simulink model "P_Control"  (R2024b)
settings: Solver=VariableStepAuto  StartTime=0.0  StopTime=time  RelTol=1e-3
values from neighbouring files (symbols this model uses):
  As = 2.15    [Data.m]
  B = (y1-y4)/2    (= 0.75)    [Data.m]
  Cd = 0.28    [Data.m]
  clockwise = 1    [Data.m]
  dd = 2    [Data.m]
  delay_Pulse_time = 1.5    [Data.m]
  derta1 = 0.5    [Data.m]
  dk = 2    [Data.m]
  Fi = Ti/r    (= 156.25)    [Data.m]
  Fz = la/(la+lb)*m*g/2    (= 2450)    [Data.m]
  id = 0.01    [Data.m]
  ik = 1    [Data.m]
  Iw = 0.5    [Data.m]
  Iz = 1600    [Data.m]
  JL = 0.08    [Data.m]
  Jm = 6.96e-6    (= 6.96e-06)    [Data.m]
  Kb = 0.0525    [Data.m]
  Kf = 1.4e-3    (= 0.0014)    [Data.m]
  Km = 0.053    [Data.m]
  L = 6.2e-4    (= 0.00062)    [Data.m]    (also in submit.m = (1-nameda1)*(1-0.015*u1*sqrt((cx^2)*(nameda1^2)+(cy^2)*((tan)
  la = x1    (= 1.25)    [Data.m]
  lb = x1    (= 1.25)    [Data.m]
  m = 1000    [Data.m]
  modeli = 1    [Data.m]
  n = 1/200    (= 0.005)    [Data.m]
  pd = 100    [Data.m]
  pk = 300    [Data.m]
  Pulse = 180    [Data.m]
  R = 2.07    [Data.m]
  r = 0.32    [Data.m]
  s_ang3 = 0    [Data.m]
  x1 = 1.25    [Data.m]
  x1_fc = 0.01    [Data.m]
  x1_jz = 0    [Data.m]
  x2 = -1.25    [Data.m]
  x2_fc = 0.05    [Data.m]
  x2_jz = 0.01    [Data.m]
  x3 = -1.25    [Data.m]
  x3_fc = 0.1    [Data.m]
  x3_jz = 0.05    [Data.m]
  x4 = 1.25    [Data.m]
  x4_fc = 0.5    [Data.m]
  x4_jz = 0.08    [Data.m]
  Xicr = 0,Yicr=10    [Data.m]
  y1 = 0.75    [Data.m]
  y2 = 0.75    [Data.m]
  y3 = -0.75    [Data.m]
  y4 = -0.75    [Data.m]
undefined symbols (not defined in the file or in its folder): Yicr
libraries: slpidlib x12
(part 2 of 2)

== system P_Control/Subsystem1/电机模型5 ==
  电流1 : Inport
  干扰 : Inport  Port=2
  Add : Sum
  Add1 : Sum  Inputs=+-
  Add2 : Sum
  Constant : Constant  Value=s_ang3
  Constant1 : Constant  Value=(Jm+n^2*JL)
  Divide : Product  Inputs=*/
  Gain3 : Gain  Gain=n*Km
  Gain4 : Gain  Gain=Kf
  Gain5 : Gain  Gain=n^2
  Integrator : Integrator
  Integrator1 : Integrator  InitialCondition=0.01
  输出转角 : Outport
  wires:
  Add2/1 -> Divide/1
  Add1/1 -> Add2/2
  Gain5/1 -> Add2/1
  Gain4/1 -> Add1/2
  Gain3/1 -> Add1/1
  Constant1/1 -> Divide/2
  Divide/1 -> Integrator1/1
  Integrator1/1 -> Gain4/1, Integrator/1
  干扰/1 -> Gain5/1
  电流1/1 -> Gain3/1
  Add/1 -> 输出转角/1
  Integrator/1 -> Add/2
  Constant/1 -> Add/1

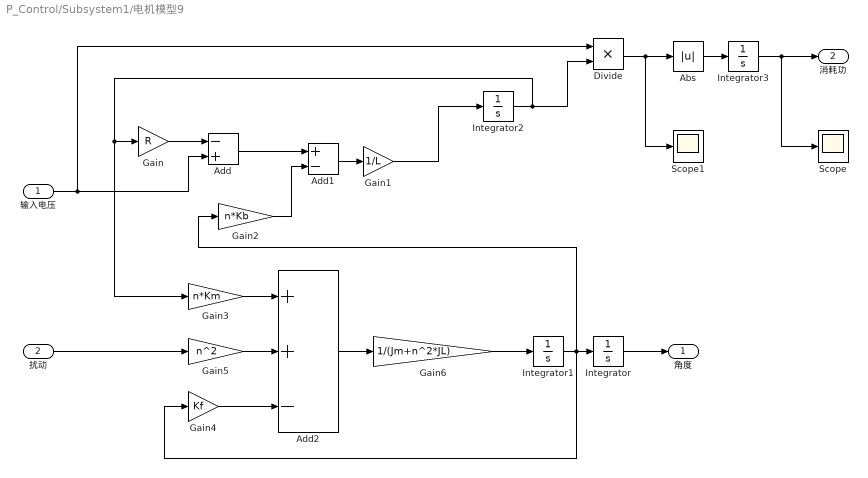
== system P_Control/Subsystem1/电机模型9 ==
  输入电压 : Inport
  扰动 : Inport  Port=2
  Abs : Abs  ZeroCross=off  SaturateOnIntegerOverflow=off
  Add : Sum  Inputs=-+
  Add1 : Sum  Inputs=+-
  Add2 : Sum  Inputs=++-
  Divide : Product  Inputs=**
  Gain : Gain  Gain=R
  Gain1 : Gain  Gain=1/L
  Gain2 : Gain  Gain=n*Kb
  Gain3 : Gain  Gain=n*Km
  Gain4 : Gain  Gain=Kf
  Gain5 : Gain  Gain=n^2
  Gain6 : Gain  Gain=1/(Jm+n^2*JL)
  Integrator{,1..3} (4 alike) : Integrator
  Scope : Scope
  Scope1 : Scope
  角度 : Outport
  消耗功 : Outport  Port=2
  wires:
  Divide/1 -> Scope1/1, Abs/1
  Gain6/1 -> Integrator1/1
  Add2/1 -> Gain6/1
  Gain4/1 -> Add2/3
  Gain5/1 -> Add2/2
  Gain3/1 -> Add2/1
  扰动/1 -> Gain5/1
  Gain1/1 -> Integrator2/1
  Add1/1 -> Gain1/1
  Gain2/1 -> Add1/2
  Add/1 -> Add1/1
  输入电压/1 -> Add/2, Divide/1
  Gain/1 -> Add/1
  Integrator2/1 -> Divide/2, Gain/1, Gain3/1
  Integrator1/1 -> Integrator/1, Gain4/1, Gain2/1
  Integrator/1 -> 角度/1
  Abs/1 -> Integrator3/1
  Integrator3/1 -> 消耗功/1, Scope/1

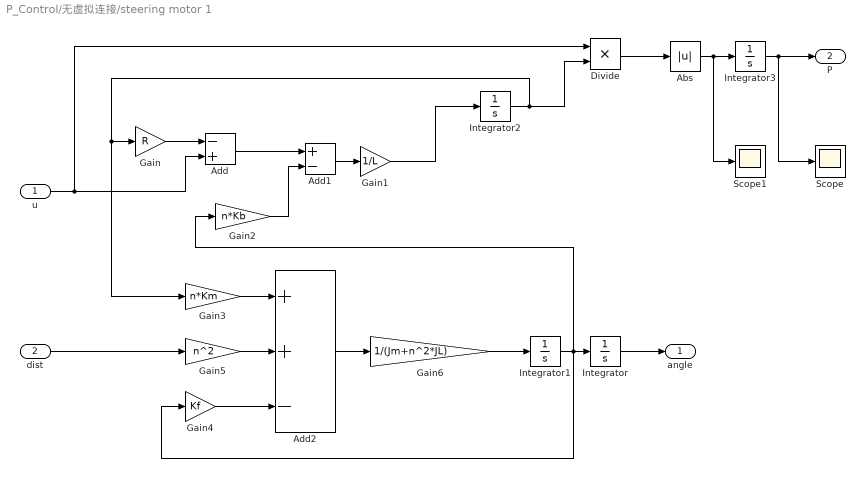
== system P_Control/无虚拟连接/steering motor 1 ==
  u : Inport
  dist : Inport  Port=2
  Abs : Abs  SaturateOnIntegerOverflow=off
  Add : Sum  Inputs=-+
  Add1 : Sum  Inputs=+-
  Add2 : Sum  Inputs=++-
  Divide : Product  Inputs=**
  Gain : Gain  Gain=R
  Gain1 : Gain  Gain=1/L
  Gain2 : Gain  Gain=n*Kb
  Gain3 : Gain  Gain=n*Km
  Gain4 : Gain  Gain=Kf
  Gain5 : Gain  Gain=n^2
  Gain6 : Gain  Gain=1/(Jm+n^2*JL)
  Integrator{,1..3} (4 alike) : Integrator
  Scope : Scope
  Scope1 : Scope
  angle : Outport
  P : Outport  Port=2
  wires:
  Integrator3/1 -> P/1, Scope/1
  Abs/1 -> Scope1/1, Integrator3/1
  Divide/1 -> Abs/1
  Gain6/1 -> Integrator1/1
  Add2/1 -> Gain6/1
  Gain4/1 -> Add2/3
  Gain5/1 -> Add2/2
  Gain3/1 -> Add2/1
  dist/1 -> Gain5/1
  Gain1/1 -> Integrator2/1
  Add1/1 -> Gain1/1
  Gain2/1 -> Add1/2
  Add/1 -> Add1/1
  u/1 -> Add/2, Divide/1
  Gain/1 -> Add/1
  Integrator2/1 -> Divide/2, Gain/1, Gain3/1
  Integrator1/1 -> Integrator/1, Gain4/1, Gain2/1
  Integrator/1 -> angle/1

== system P_Control/无虚拟连接/steering motor 2 ==
  u : Inport
  dist : Inport  Port=2
  Abs : Abs  SaturateOnIntegerOverflow=off
  Add : Sum  Inputs=-+
  Add1 : Sum  Inputs=+-
  Add2 : Sum  Inputs=++-
  Divide : Product  Inputs=**
  Gain : Gain  Gain=R
  Gain1 : Gain  Gain=1/L
  Gain2 : Gain  Gain=n*Kb
  Gain3 : Gain  Gain=n*Km
  Gain4 : Gain  Gain=Kf
  Gain5 : Gain  Gain=n^2
  Gain6 : Gain  Gain=1/(Jm+n^2*JL)
  Integrator{,1..3} (4 alike) : Integrator
  Scope : Scope
  angle : Outport
  P : Outport  Port=2
  wires:
  Integrator3/1 -> P/1, Scope/1
  Abs/1 -> Integrator3/1
  Divide/1 -> Abs/1
  Gain6/1 -> Integrator1/1
  Add2/1 -> Gain6/1
  Gain4/1 -> Add2/3
  Gain5/1 -> Add2/2
  Gain3/1 -> Add2/1
  dist/1 -> Gain5/1
  Gain1/1 -> Integrator2/1
  Add1/1 -> Gain1/1
  Gain2/1 -> Add1/2
  Add/1 -> Add1/1
  u/1 -> Add/2, Divide/1
  Gain/1 -> Add/1
  Integrator2/1 -> Divide/2, Gain/1, Gain3/1
  Integrator1/1 -> Integrator/1, Gain4/1, Gain2/1
  Integrator/1 -> angle/1

== system P_Control/无虚拟连接/steering motor 3 ==
  u : Inport
  dist : Inport  Port=2
  Abs : Abs  SaturateOnIntegerOverflow=off
  Add : Sum  Inputs=-+
  Add1 : Sum  Inputs=+-
  Add2 : Sum  Inputs=++-
  Divide : Product  Inputs=**
  Gain : Gain  Gain=R
  Gain1 : Gain  Gain=1/L
  Gain2 : Gain  Gain=n*Kb
  Gain3 : Gain  Gain=n*Km
  Gain4 : Gain  Gain=Kf
  Gain5 : Gain  Gain=n^2
  Gain6 : Gain  Gain=1/(Jm+n^2*JL)
  Integrator{,1..3} (4 alike) : Integrator
  Scope : Scope
  angle : Outport
  P : Outport  Port=2
  wires:
  Integrator/1 -> angle/1
  Integrator1/1 -> Gain2/1, Gain4/1, Integrator/1
  Integrator2/1 -> Gain3/1, Gain/1, Divide/2
  Gain/1 -> Add/1
  u/1 -> Divide/1, Add/2
  Add/1 -> Add1/1
  Gain2/1 -> Add1/2
  Add1/1 -> Gain1/1
  Gain1/1 -> Integrator2/1
  dist/1 -> Gain5/1
  Gain3/1 -> Add2/1
  Gain5/1 -> Add2/2
  Gain4/1 -> Add2/3
  Add2/1 -> Gain6/1
  Gain6/1 -> Integrator1/1
  Divide/1 -> Abs/1
  Abs/1 -> Integrator3/1
  Integrator3/1 -> P/1, Scope/1

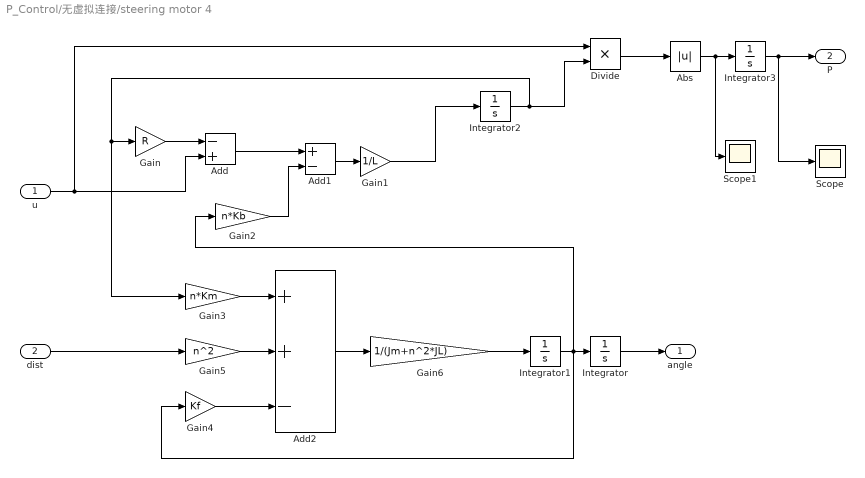
== system P_Control/无虚拟连接/steering motor 4 ==
  u : Inport
  dist : Inport  Port=2
  Abs : Abs  SaturateOnIntegerOverflow=off
  Add : Sum  Inputs=-+
  Add1 : Sum  Inputs=+-
  Add2 : Sum  Inputs=++-
  Divide : Product  Inputs=**
  Gain : Gain  Gain=R
  Gain1 : Gain  Gain=1/L
  Gain2 : Gain  Gain=n*Kb
  Gain3 : Gain  Gain=n*Km
  Gain4 : Gain  Gain=Kf
  Gain5 : Gain  Gain=n^2
  Gain6 : Gain  Gain=1/(Jm+n^2*JL)
  Integrator{,1..3} (4 alike) : Integrator
  Scope : Scope
  Scope1 : Scope
  angle : Outport
  P : Outport  Port=2
  wires:
  Integrator/1 -> angle/1
  Integrator1/1 -> Gain2/1, Gain4/1, Integrator/1
  Integrator2/1 -> Gain3/1, Gain/1, Divide/2
  Gain/1 -> Add/1
  u/1 -> Divide/1, Add/2
  Add/1 -> Add1/1
  Gain2/1 -> Add1/2
  Add1/1 -> Gain1/1
  Gain1/1 -> Integrator2/1
  dist/1 -> Gain5/1
  Gain3/1 -> Add2/1
  Gain5/1 -> Add2/2
  Gain4/1 -> Add2/3
  Add2/1 -> Gain6/1
  Gain6/1 -> Integrator1/1
  Divide/1 -> Abs/1
  Abs/1 -> Scope1/1, Integrator3/1
  Integrator3/1 -> P/1, Scope/1

== matlab function P_Control/Subsystem/前后轮X,Y方向力 ==
  data: F1 input; Fx1 output; F2 input; F3 input; F4 input; f1 input; f2 input; f3 input; f4 input; deta1 input; deta2 input; Fy1 output; Fx2 output; Fy2 output; deta3 input; deta4 input; Fx3 output; Fy3 output; Fx4 output; Fy4 output
function [Fx1,Fy1,Fx2,Fy2,Fx3,Fy3,Fx4,Fy4]= fcn(F1,F2, F3,F4,f1,f2,f3,f4,deta1,deta2,deta3,deta4)

Fx1=F1*cos(deta1)-f1*sin(deta1);
Fy1=F1*sin(deta1)+f1*cos(deta1);


Fx2=F2*cos(deta2)-f2*sin(deta2);
Fy2=F2*sin(deta2)+f2*cos(deta2);

Fx3=F3*cos(deta3)-f3*sin(deta3);
Fy3=F3*sin(deta3)+f3*cos(deta3);

Fx4=F4*cos(deta4)-f4*sin(deta4);
Fy4=F4*sin(deta4)+f4*cos(deta4);

== matlab function P_Control/Subsystem/横向速度计算 ==
  data: Fy1 input; dVy output; Fy2 input; Fy3 input; Fy4 input; m input; w input; Vx input
function dVy= fcn(Fy1,Fy2,Fy3,Fy4,m,w,Vx)


dVy=(Fy2+Fy1+Fy1+Fy2)/m-Vx*w;

== matlab function P_Control/Subsystem/横摆角速度计算 ==
  data: Fx1 input; Fx2 input; Fx3 input; Fx4 input; Fy1 input; dW output; Fy2 input; Fy3 input; Fy4 input; Iz input; la input; lb input; B input
function dW= fcn(Fx1,Fx2,Fx3,Fx4,Fy1,Fy2,Fy3,Fy4,Iz,la,lb,B)

% dW=((Fy4+Fy1)*la-(Fy2+Fy3)*lb)/Iz;

dW=((Fy4+Fy1)*la-(Fy2+Fy3)*lb+(Fx4+Fx3)*B-(Fx1+Fx2)*B)/Iz;

== matlab function P_Control/Subsystem/纵向速度计算 ==
  data: Fx1 input; dVx output; Fx2 input; Fx3 input; Fx4 input; m input; w input; Vy input
function dVx= fcn(Fx1,Fx2,Fx3,Fx4,m,w,Vy)


dVx=(Fx1+Fx2+Fx3+Fx4)/m+Vy*w;

== matlab function P_Control/Subsystem/魔术轮胎公式 ==
  data: a11 input; a22 input; a33 input; a44 input; f1 output; Fz input; f2 output; f3 output; f4 output
function [f1,f2,f3,f4] = fcn(a11,a22,a33,a44,Fz)

a1=-22.1;
a2=1011;
a3=1078;
a4=1.82;
a5=0.208;
a6=0;
a7=-0.354;
a8=0.707;
a9=0.028;
a10=0;
a12=0.022;
C=1.3;
D=a1*Fz^2+a2*Fz;
BCD=a3*sin(a4*atan(a5*Fz));
B=BCD/(C*D);
E=a6*Fz^2+a7*Fz+a8;

f1=-D*sin(C*atan(B*a11-E*(B*a11-atan(B*a11))));
f2=-D*sin(C*atan(B*a22-E*(B*a22-atan(B*a22))));
f3=-D*sin(C*atan(B*a33-E*(B*a33-atan(B*a33))));
f4=-D*sin(C*atan(B*a44-E*(B*a44-atan(B*a44))));

== matlab function P_Control/无虚拟连接/alpha ==
  data: Vx input; a1 output; Vy input; w input; deta1 input; deta2 input; deta3 input; deta4 input; la input; lb input; a2 output; B input; a3 output; a4 output
function [a1,a2,a3,a4] = fcn(Vx,Vy,w,deta1,deta2,deta3,deta4,la,lb,B)


a1=atan((Vy+la*w)/(Vx-w*B))-deta1;
a2=atan((Vy-lb*w)/(Vx-w*B))-deta2;
a3=atan((Vy-la*w)/(Vx+w*B))-deta3;
a4=atan((Vy+la*w)/(Vx+w*B))-deta4;

== matlab function P_Control/无虚拟连接/Forces in X and Y directions of front and rear wheels ==
  data: F1 input; Fx1 output; F2 input; F3 input; F4 input; f1 input; f2 input; f3 input; f4 input; deta1 input; deta2 input; Fy1 output; Fx2 output; Fy2 output; deta3 input; deta4 input; Fx3 output; Fy3 output; Fx4 output; Fy4 output
function [Fx1,Fy1,Fx2,Fy2,Fx3,Fy3,Fx4,Fy4]= fcn(F1,F2, F3,F4,f1,f2,f3,f4,deta1,deta2,deta3,deta4)

Fx1=F1*cos(deta1)-f1*sin(deta1);
Fy1=F1*sin(deta1)+f1*cos(deta1);


Fx2=F2*cos(deta2)+f2*sin(deta2);
Fy2=-F2*sin(deta2)+f2*cos(deta2);

Fx3=F3*cos(deta3)+f3*sin(deta3);
Fy3=-F3*sin(deta3)+f3*cos(deta3);

Fx4=F4*cos(deta4)-f4*sin(deta4);
Fy4=F4*sin(deta4)+f4*cos(deta4);

== matlab function P_Control/Subsystem1/虚拟连接计算角度3 ==
  data: deta1 input; angout output; deta2 input; deta3 input; deta4 input
function angout = fcn(deta1,deta2,deta3,deta4)

deta=[deta1,deta2,deta3,deta4];
angout=[0,0,0,0];

x=[2,-2,-2,2];
y=[1,1,-1,-1];
a=[0,0,0,0];
b=[0,0,0,0];
a_new=[0,0,0,0];
b_new=[0,0,0,0];

A1=0;
A2=0;
A3=0;
A4=0;
A5=0;

% if (deta(1)~=0) && (deta(2)~=0) && (deta(3)~=0) && (deta(4)~=0)
% 
%         for i =1:4
%             a(i)=tan(deta(i)+pi/2);
%             b(i)=y(i)-a(i)*x(i);
%         end
%         Xf=-(b(1)-b(4))/(a(1)-a(4));
%         Yf=(a(1)*b(4)-a(4)*b(1))/(a(1)-a(4));
% 
%         Kf=Yf/(Xf-x(1));
%         bf=-Yf*x(1)/(Xf-x(1));
% 
%         Xr=-(b(2)-b(3))/(a(2)-a(3));
%         Yr=(a(2)*b(3)-a(3)*b(2))/(a(2)-a(3));
% 
%         Kr=Yr/(Xr-x(2));
%         br=-Yr*x(2)/(Xr-x(2));
% 
%         Xicr_c=-(bf-br)/(Kf-Kr);
%         Yicr_c=(Kf*br-Kr*bf)/(Kf-Kr);
%         for i=1:4
%             k=sign(deta(i)-atan2(y(i)-Yicr_c,x(i)-Xicr_c));
%             angout(i)=atan2(k*(x(i)-Xicr_c),-k*(y(i)-Yicr_c));
%         end
% 
% elseif ((deta(1)==0) || (deta(4)==0)) && (deta(2)~=0) && (deta(3)~=0)
%     for i =2:3
%         a(i)=tan(deta(i)+pi/2);
%         b(i)=y(i)-a(i)*x(i);
%     end
%     Xr=-(b(2)-b(3))/(a(2)-a(3));
%     Yr=(a(2)*b(3)-a(3)*b(2))/(a(2)-a(3));
%     Kr=Yr/(Xr-x(2));
%     br=-Yr*x(2)/(Xr-x(2));
%     Xicr_c=x(1);
%     Yicr_c=Kr*x(1)+br;
%     for i=1:4
%         k=sign(deta(i)-atan2(y(i)-Yicr_c,x(i)-Xicr_c));
%         angout(i)=atan2(k*(x(i)-Xicr_c),-k*(y(i)-Yicr_c));
%     end
% 
% elseif ((deta(2)==0) || (deta(3)==0)) && (deta(1)~=0) && (deta(4)~=0)
%     a(1)=tan(deta(1)+pi/2);
%     b(1)=y(1)-a(1)*x(1);
%     a(2)=tan(deta(2)+pi/2);
%     b(2)=y(2)-a(2)*x(2);
%     Xf=-(b(1)-b(4))/(a(1)-a(4));
%     Yf=(a(1)*b(4)-a(4)*b(1))/(a(1)-a(4));
%     Kf=Yf/(Xf-x(1));
%     bf=-Yf*x(1)/(Xf-x(1));
%     Xicr_c=x(2);
%     Yicr_c=Kf*x(2)+bf;
%     for i=1:4
%       k=sign(deta(i)-atan2(y(i)-Yicr_c,x(i)-Xicr_c));
%       angout(i)=atan2(k*(x(i)-Xicr_c),-k*(y(i)-Yicr_c));
%     end
% end



if (deta(1)~=0) && (deta(2)~=0) && (deta(3)~=0) && (deta(4)~=0)

        for i =1:4
            a(i)=tan(deta(i)+pi/2);
            b(i)=y(i)-a(i)*x(i);
        end
        X1=-(b(1)-b(4))/(a(1)-a(4));
        Y1=(a(1)*b(4)-a(4)*b(1))/(a(1)-a(4));

        K1=Y1/(X1-x(1));
        b1=-Y1*x(1)/(X1-x(1));

        X2=-(b(2)-b(3))/(a(2)-a(3));
        Y2=(a(2)*b(3)-a(3)*b(2))/(a(2)-a(3));

        K2=Y2/(X2-x(2));
        b2=-Y2*x(2)/(X2-x(2));
        
        X3=-(b(1)-b(2))/(a(1)-a(2));
        Y3=(a(1)*b(2)-a(2)*b(1))/(a(1)-a(2));

        K3=(Y3-y(1))/X3;
        b3=y(1);

        X4=-(b(4)-b(3))/(a(4)-a(3));
        Y4=(a(4)*b(3)-a(3)*b(4))/(a(4)-a(3));

        K4=(Y4-y(4))/X4;
        b4=y(4);
        a_new(1)=K1;a_new(2)=K2;a_new(3)=K3;a_new(4)=K4;
        b_new(1)=b1;b_new(2)=b2;b_new(3)=b3;b_new(4)=b4;

        for i=1:4
         A1=A1+2*a_new(i)^2/(a_new(i)^2+1);
         A2=A2+2*a_new(i)/(a_new(i)^2+1);
         A3=A3+2*a_new(i)*b_new(i)/(a_new(i)^2+1);
         A4=A4+2/(a_new(i)^2+1);
         A5=A5+2*b_new(i)/(a_new(i)^2+1);
        end

        Xicr_c=(A2*A5-A3*A4)/(A1*A4-A2^2)
        Yicr_c=(A1*A5-A3*A2)/(A1*A4-A2^2)

        for i=1:4
            k=sign(deta(i)-atan2(y(i)-Yicr_c,x(i)-Xicr_c));
            angout(i)=atan2(k*(x(i)-Xicr_c),-k*(y(i)-Yicr_c));
        end
end

== matlab function P_Control/无虚拟连接/Omega ==
  data: Fx1 input; Fx2 input; Fx3 input; Fx4 input; Fy1 input; dW output; Fy2 input; Fy3 input; Fy4 input; Iz input; la input; lb input; B input
function dW= fcn(Fx1,Fx2,Fx3,Fx4,Fy1,Fy2,Fy3,Fy4,Iz,la,lb,B)

% dW=((Fy4+Fy1)*la-(Fy2+Fy3)*lb)/Iz;

dW=((Fy4+Fy1)*la-(Fy2+Fy3)*lb+(Fx4+Fx3)*B-(Fx1+Fx2)*B)/Iz;

== matlab function P_Control/无虚拟连接/ target steering angle ==
  data: Yicr input; deta4 output; deta1 output; deta3 output; deta2 output; Xicr input
function [deta4,deta1,deta3,deta2] = fcn(Yicr,Xicr)

x=[1.25,-1.25,-1.25,1.25];
y=[0.75,0.75,-0.75,-0.75];

if Yicr>0
    u1=1
    deta1=atan2(u1*(x(1)-Xicr),-u1*(y(1)-Yicr));
    deta2=atan2(u1*(x(2)-Xicr),-u1*(y(2)-Yicr));
    deta3=atan2(u1*(x(3)-Xicr),-u1*(y(3)-Yicr));
    deta4=atan2(u1*(x(4)-Xicr),-u1*(y(4)-Yicr));
else
    u1=-1
    deta1=atan2(u1*(x(1)-Xicr),-u1*(y(1)-Yicr));
    deta2=atan2(u1*(x(2)-Xicr),-u1*(y(2)-Yicr));
    deta3=atan2(u1*(x(3)-Xicr),-u1*(y(3)-Yicr));
    deta4=atan2(u1*(x(4)-Xicr),-u1*(y(4)-Yicr));
end

== matlab function P_Control/无虚拟连接/Vx ==
  data: Fx1 input; dVx output; Fx2 input; Fx3 input; Fx4 input; m input; w input; Vy input; vx input; Cd input; As input
function dVx= fcn(Fx1,Fx2,Fx3,Fx4,m,w,Vy,vx,Cd,As)


dVx=(Fx1+Fx2+Fx3+Fx4-As*Cd*vx^2/21.15)/m+Vy*w;

== matlab function P_Control/无虚拟连接/lambda ==
  data: u1 input; lambda1 output; u2 input; u3 input; u4 input; Vx input; lambda2 output; lambda3 output; lambda4 output
function [lambda1,lambda2,lambda3,lambda4] = fcn(u1,u2,u3,u4,Vx)

lambda1=(Vx-u1)/Vx;
lambda2=(Vx-u2)/Vx;
lambda3=(Vx-u3)/Vx;
lambda4=(Vx-u4)/Vx;

== matlab function P_Control/Subsystem/MATLAB Function ==
  data: vx input; m input; vy input; y output
function y = fcn(vx,m,vy)

y = 1/2*(sqrt(vx^2+vy^2))^2*m;

== matlab function P_Control/无虚拟连接/MATLAB Function ==
  data: vx input; y output; m input; vy input; V output
function [y,V] = fcn(vx,m,vy)

y = 1/2*(sqrt(vx^2+vy^2))^2*m;
V=sqrt(vx^2+vy^2);

== matlab function P_Control/无虚拟连接/v of the  wheel ==
  data: deta1 input; u1 output; deta2 input; deta3 input; deta4 input; la input; lb input; Vx input; Vy input; w input; B input; u2 output; u3 output; u4 output
function [u1,u2,u3,u4] = fcn(deta1,deta2,deta3,deta4,la,lb,Vx,Vy,w,B)

u1=(Vx-w*B)*cos(deta1)+(Vy+w*la)*sin(deta1);
u2=(Vx-w*B)*cos(deta2)+(Vy-w*lb)*sin(deta2);
u3=(Vx+w*B)*cos(deta3)+(Vy-w*lb)*sin(deta3);
u4=(Vx+w*B)*cos(deta4)+(Vy+w*la)*sin(deta4);

== matlab function P_Control/无虚拟连接/energy loss caused by lateral slip of wheel ==
  data: nameda1 input; P1 output; nameda2 input; nameda3 input; nameda4 input; u1 input; u2 input; u3 input; u4 input; Fx1 input; Fx2 input; Fx3 input; Fx4 input; P2 output; P3 output; P4 output
function [P1,P2,P3,P4] = fcn(nameda1,nameda2,nameda3,nameda4,u1,u2,u3,u4,Fx1,Fx2,Fx3,Fx4)

P1=Fx1*nameda1*u1;
P2=Fx2*nameda2*u2;
P3=Fx3*nameda3*u3;
P4=Fx4*nameda4*u4;

== matlab function P_Control/无虚拟连接/Total kinetic energy of the wheels ==
  data: u1 input; Ew output; u2 input; u3 input; u4 input; Iw input; r input
function Ew = fcn(u1,u2,u3,u4,Iw,r)

Ew=1/2*Iw*((u1/r)^2+(u2/r)^2+(u3/r)^2+(u4/r)^2)

== matlab function P_Control/无虚拟连接/dugoff1  ==
  data: Fz input; u input; nameda1 input; alpha1 input; f1 output; u1 input
function f1 = tire(Fz,u,nameda1,alpha1,u1)
nameda1 = -nameda1;
cx = -4;
cy = -20;
L = (1-nameda1)*(1-0.015*u1*sqrt((cx^2)*(nameda1^2)+(cy^2)*((tan(alpha1))^2)))/(2*sqrt((cx^2)*(nameda1^2)+(cy^2)*((tan(alpha1))^2)));
if L<1
    fL = L*(2-L);
else
    fL = 1;
end
Fx0 = Fz*cx*nameda1*fL/(1-nameda1);
Fy0 = Fz*cy*tan(alpha1)*fL/(1-nameda1);
Fx = u*Fx0;
f1 = u*Fy0;

== matlab function P_Control/Subsystem/虚拟连接计算角度2 ==
  data: deta1 input; angout output; deta2 input; deta3 input; deta4 input
function angout = fcn(deta1,deta2,deta3,deta4)

deta=[deta1,deta2,deta3,deta4];
angout=[0,0,0,0];

x=[1.25,-1.25,-1.25,1.25];
y=[0.75,0.75,-0.75,-0.75];
a=[0,0,0,0];
b=[0,0,0,0];

if (deta(1)~=0) && (deta(2)~=0) && (deta(3)~=0) && (deta(4)~=0)

        for i =1:4
            a(i)=tan(deta(i)+pi/2)
            b(i)=y(i)-a(i)*x(i)
        end
        Xf=-(b(1)-b(4))/(a(1)-a(4));
        Yf=(a(1)*b(4)-a(4)*b(1))/(a(1)-a(4));
        Kf=Yf/(Xf-x(1));
        bf=-Yf*x(1)/(Xf-x(1));
        
        Xr=-(b(2)-b(3))/(a(2)-a(3));
        Yr=(a(2)*b(3)-a(3)*b(2))/(a(2)-a(3));
        
        Kr=Yr/(Xr-x(2));
        br=-Yr*x(2)/(Xr-x(2));
        
        Xicr_c=-(bf-br)/(Kf-Kr);
        Yicr_c=(Kf*br-Kr*bf)/(Kf-Kr);
        for i=1:4
            k=sign(deta(i)-atan2(y(i)-Yicr_c,x(i)-Xicr_c));
            angout(i)=atan2(k*(x(i)-Xicr_c),-k*(y(i)-Yicr_c));
        end

elseif ((deta(1)==0) || (deta(4)==0)) && (deta(2)~=0) && (deta(3)~=0)
    for i =2:3
        a(i)=tan(deta(i)+pi/2);
        b(i)=y(i)-a(i)*x(i);
    end
    Xr=-(b(2)-b(3))/(a(2)-a(3));
    Yr=(a(2)*b(3)-a(3)*b(2))/(a(2)-a(3));
    Kr=Yr/(Xr-x(2));
    br=-Yr*x(2)/(Xr-x(2));
    Xicr_c=x(1);
    Yicr_c=Kr*x(1)+br;
    for i=1:4
        k=sign(deta(i)-atan2(y(i)-Yicr_c,x(i)-Xicr_c));
        angout(i)=atan2(k*(x(i)-Xicr_c),-k*(y(i)-Yicr_c));
    end

elseif ((deta(2)==0) || (deta(3)==0)) && (deta(1)~=0) && (deta(4)~=0)
    a(1)=tan(deta(1)+pi/2);
    b(1)=y(1)-a(1)*x(1);
    a(2)=tan(deta(2)+pi/2);
    b(2)=y(2)-a(2)*x(2)
    Xf=-(b(1)-b(4))/(a(1)-a(4));
    Yf=(a(1)*b(4)-a(4)*b(1))/(a(1)-a(4));
    Kf=Yf/(Xf-x(1));
    bf=-Yf*x(1)/(Xf-x(1));
    Xicr_c=x(2);
    Yicr_c=Kf*x(2)+bf;
    for i=1:4
      k=sign(deta(i)-atan2(y(i)-Yicr_c,x(i)-Xicr_c));
      angout(i)=atan2(k*(x(i)-Xicr_c),-k*(y(i)-Yicr_c));
    end
end

== matlab function P_Control/无虚拟连接/dugoff2 ==
  data: Fz input; u input; nameda2 input; alpha2 input; f2 output; u2 input
function f2 = tire(Fz,u,nameda2,alpha2,u2)
nameda2 = -nameda2;
cx = -4;
cy = -20;
L = (1-nameda2)*(1-0.015*u2*sqrt((cx^2)*(nameda2^2)+(cy^2)*((tan(alpha2))^2)))/(2*sqrt((cx^2)*(nameda2^2)+(cy^2)*((tan(alpha2))^2)));
if L<1
    fL = L*(2-L);
else
    fL = 1;
end
Fx0 = Fz*cx*nameda2*fL/(1-nameda2);
Fy0 = Fz*cy*tan(alpha2)*fL/(1-nameda2);
Fx = u*Fx0;
f2 = u*Fy0;

== matlab function P_Control/无虚拟连接/dugoff3 ==
  data: Fz input; u input; nameda3 input; alpha3 input; f3 output; u3 input
function f3 = tire(Fz,u,nameda3,alpha3,u3)
nameda3 = -nameda3;
cx = -4;
cy = -20;
L = (1-nameda3)*(1-0.015*u3*sqrt((cx^2)*(nameda3^2)+(cy^2)*((tan(alpha3))^2)))/(2*sqrt((cx^2)*(nameda3^2)+(cy^2)*((tan(alpha3))^2)));
if L<1
    fL = L*(2-L);
else
    fL = 1;
end
Fx0 = Fz*cx*nameda3*fL/(1-nameda3);
Fy0 = Fz*cy*tan(alpha3)*fL/(1-nameda3);
Fx = u*Fx0;
f3 = u*Fy0;

== matlab function P_Control/无虚拟连接/dugoff4 ==
  data: Fz input; u input; nameda4 input; alpha4 input; f4 output; u4 input
function f4 = tire(Fz,u,nameda4,alpha4,u4)
nameda4 = -nameda4;
cx = -4;
cy = -20;
L = (1-nameda4)*(1-0.015*u4*sqrt((cx^2)*(nameda4^2)+(cy^2)*((tan(alpha4))^2)))/(2*sqrt((cx^2)*(nameda4^2)+(cy^2)*((tan(alpha4))^2)));
if L<1
    fL = L*(2-L);
else
    fL = 1;
end
Fx0 = Fz*cx*nameda4*fL/(1-nameda4);
Fy0 = Fz*cy*tan(alpha4)*fL/(1-nameda4);
Fx = u*Fx0;
f4 = u*Fy0;

== matlab function P_Control/无虚拟连接/Vy ==
  data: Fy1 input; dVy output; Fy2 input; Fy3 input; Fy4 input; m input; w input; Vx input
function dVy= fcn(Fy1,Fy2,Fy3,Fy4,m,w,Vx)


dVy=(Fy2+Fy1+Fy3+Fy4)/m-Vx*w;

== matlab function P_Control/无虚拟连接/energy loss by longitudinal slip of wheel ==
  data: Fy1 input; Ph1 output; Fy2 input; Fy3 input; Fy4 input; Vx input; a1 input; a2 input; a3 input; a4 input; Ph2 output; Ph3 output; Ph4 output
function [Ph1,Ph2,Ph3,Ph4] = fcn(Fy1,Fy2,Fy3,Fy4,Vx,a1,a2,a3,a4)

Ph1=-Fy1*Vx*a1;
Ph2=-Fy2*Vx*a2;
Ph3=-Fy3*Vx*a3;
Ph4=-Fy4*Vx*a4;

== matlab function P_Control/Subsystem/Subsystem4/MATLAB Function ==
  data: derta4 input; u1 output; u2 output
function [u1,u2] = fcn(derta4)

if derta4>0
    u1=1
else
    u1=-1
end
u2=-u1

== matlab function P_Control/Subsystem/侧偏角计算 ==
  data: Vx input; a1 output; Vy input; w input; deta1 input; deta2 input; deta3 input; deta4 input; la input; lb input; a2 output; B input; a3 output; a4 output
function [a1,a2,a3,a4] = fcn(Vx,Vy,w,deta1,deta2,deta3,deta4,la,lb,B)


a1=atan((Vy+la*w)/(Vx-w*B))-deta1;
a2=atan((Vy-lb*w)/(Vx-w*B))-deta2;
a3=atan((Vy-la*w)/(Vx+w*B))-deta3;
a4=atan((Vy+la*w)/(Vx+w*B))-deta4;
